simulink model "empc_aircraft"  (R2023a)
settings: Solver=ode45  StartTime=0.0  StopTime=5  RelTol=1e-3
values from neighbouring files (symbols this model uses):
  A = [-0.0151 -60.5651 0 -32.174 ... (first row only)    [empcaircraft1.m]
  B = [-2.516 -13.136 ... (first row only)    [empcaircraft1.m]
  C = [0 1 0 0 ... (first row only)    [empcaircraft1.m]
  D = [0 0 ... (first row only)    [empcaircraft1.m]
  x0 = zeros(4,1)    [empcaircraft1.m]
libraries: mpclib x1
settings Model: ExtModeTrigMode=oneshot  Creator=The MathWorks, Inc.  LastModifiedBy=The MathWorks, Inc.
settings SolverCC: AlgebraicLoopSolver=TrustRegion  MaxZcPerStep=1
settings DataIOCC: SaveFormat=Array  SaveOutput=off  SignalLogging=off  DSMLogging=off  SaveTime=off  ReturnWorkspaceOutputs=off  SignalLoggingName=sigsOut
settings OptimizationCC: BooleanDataType=off  ExpressionDepthLimit=2147483647  InitFltsAndDblsToZero=on  LifeSpan=inf
settings DebuggingCC: SaveWithParameterizedLinksMsg=none  UnderspecifiedInitializationDetection=Classic  MergeDetectMultiDrivingBlocksExec=none  CheckExecutionContextPreStartOutputMsg=on  SignalResolutionControl=TryResolveAllWithWarning  MultiTaskDSMMsg=warning  MultiTaskCondExecSysMsg=none  IntegerOverflowMsg=none  FcnCallInpInsideContextMsg=warning  UnconnectedInputMsg=warning  UnconnectedOutputMsg=warning  UnconnectedLineMsg=warning  StateNameClashWarn=warning  SFUnexpectedBacktrackingDiag=warning  SFNoUnconditionalDefaultTransitionDiag=warning  SFExecutionAtInitializationDiag=none  IntegerSaturationMsg=none  ArithmeticOperatorsInVariantConditions=warning
settings HardwareCC: ProdBitPerPointer=32  ProdBitPerSizeT=32  ProdBitPerPtrDiffT=32  ProdLargestAtomicFloat=None  ProdIntDivRoundTo=Undefined  ProdEndianess=Unspecified  ProdWordSize=32  ProdHWDeviceType=32-bit Generic  TargetUnknown=on
settings ModelReferenceCC: EnableRefExpFcnMdlSchedulingChecks=on  PropagateSignalLabelsOutOfModel=off
settings SFSimCC: SimUseLocalCustomCode=off  CustomCodeUndefinedFunction=UseInterfaceOnly
settings RTWCC: RTWUseLocalCustomCode=off  DLArmComputeVersion=19.05
settings CodeAppCC: StateflowObjectComments=on
settings GRTTargetCC: TargetFcnLib=ansi_tfl_tmw.mat  TargetLangStandard=C89/C90 (ANSI)  CombineOutputUpdateFcns=off  GRTInterface=on
settings ConfigComp: CovMetricSettings=dw  CovSaveCumulativeToWorkspaceVar=on  CovSaveSingleToWorkspaceVar=on  CovExternalEMLEnable=off  CovSFcnEnable=off

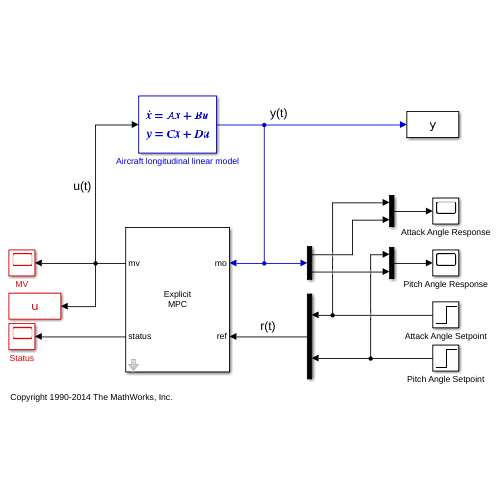
[thumbnail: Simulink's stored preview of the top-level diagram]
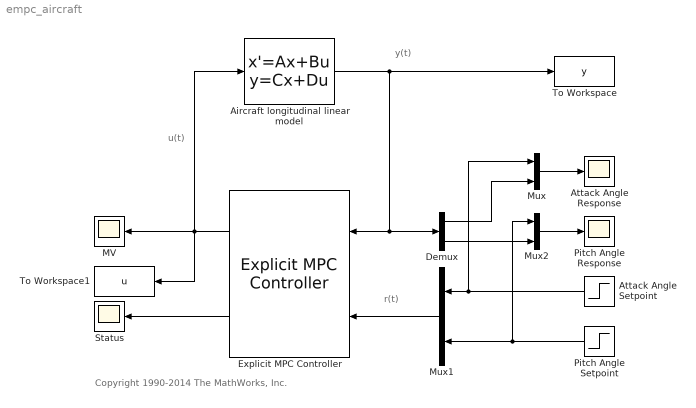
== system empc_aircraft ==
  note: u(t)
  note: y(t)
  note: r(t)
  note: Copyright 1990-2014 The MathWorks, Inc.
  Aircraft longitudinal linear model : StateSpace  A=A  B=B  C=C  D=D  InitialCondition=x0
  Attack Angle Response : Scope
  Attack Angle Setpoint : Step  After=0.1  SampleTime=0
  Demux : Demux  Outputs=2
  Explicit MPC Controller : mpclib/Explicit MPC Controller  SCDEnableBlockLinearizationSpecification=on  empcobj=empcobjSimplified  is_multiple=0  enable_value=0  return_u0=off  md_inport=off  mv_inport=off  return_status=on  return_region=off  return_state=off  state_inport=off  BlockDataType=double  SampleTimeInherited=off  switch_inport=off
  MV : Scope
  Mux : Mux  Inputs=2
  Mux1 : Mux  Inputs=2
  Mux2 : Mux  Inputs=2
  Pitch Angle Response : Scope
  Pitch Angle Setpoint : Step  Time=2  After=2  SampleTime=0
  Status : Scope
  To Workspace : ToWorkspace  VariableName=y  SampleTime=-1
  To Workspace1 : ToWorkspace  VariableName=u  SampleTime=-1
  wires:
  Aircraft longitudinal linear model/1 -> To Workspace/1, Explicit MPC Controller/1, Demux/1
  Mux/1 -> Attack Angle Response/1
  Explicit MPC Controller/1 -> To Workspace1/1, MV/1, Aircraft longitudinal linear model/1
  Attack Angle Setpoint/1 -> Mux/1, Mux1/1
  Pitch Angle Setpoint/1 -> Mux1/2, Mux2/1
  Mux1/1 -> Explicit MPC Controller/2
  Demux/1 -> Mux/2
  Mux2/1 -> Pitch Angle Response/1
  Demux/2 -> Mux2/2
  Explicit MPC Controller/2 -> Status/1
